simulink model "W04_4_inner_loop_offline"  (R2024b)
settings: Solver=ode4  StartTime=0.0  StopTime=40  FixedStep=0.05  RelTol=1e-3
values from neighbouring files (symbols this model uses):
  animate = 1    [W04_setup.m]
  Kd_psi = -400    [W04_setup.m]
  Ki_psi = 0    [W04_setup.m]
  Kp_psi = 800    [W04_setup.m]
  N_max = 500    [W04_setup.m]
  psi_ref_deg = 45    [W04_setup.m]
  use_ssa = 1    [W04_setup.m]
undefined symbols (not defined in the file or in its folder): DiscIntNeverNeededParam
libraries: slpidlib x1
settings Model: Creator=admin  LastModifiedBy=admin

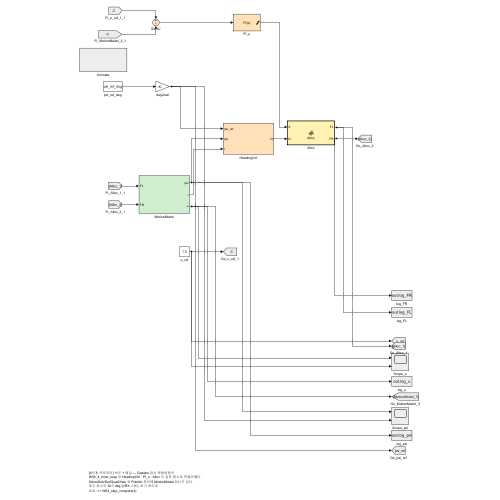
[thumbnail: Simulink's stored preview of the top-level diagram]
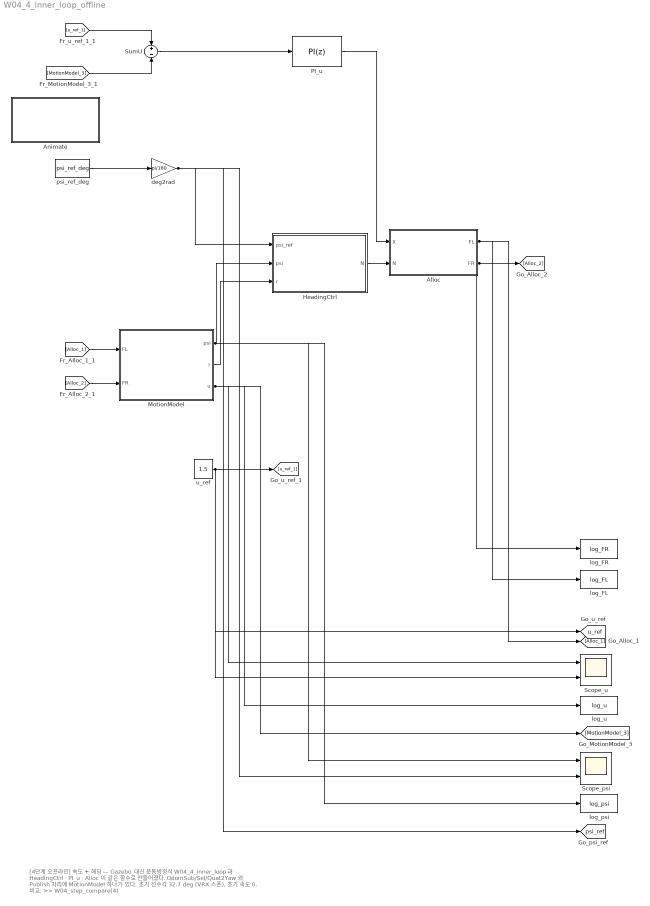
== system W04_4_inner_loop_offline ==
  note: [4단계 오프라인] 속도 + 헤딩 — Gazebo 대신 운동방정식
      | W04_4_inner_loop 과 HeadingCtrl · PI_u · Alloc 이 같은 함수로 만들어졌다.
      | OdomSub/Sel/Quat2Yaw 와 Publish 자리에 MotionModel 하나가 있다.
      | 초기 선수각 32.7 deg (VRX 스폰), 초기 속도 0.
      | 비교: >> W04_step_compare(4)
  Alloc : MATLAB Function  TreatAsAtomicUnit=on
  Animate : Subsystem
  HeadingCtrl : Subsystem
  MotionModel : Subsystem
  PI_u : slpidlib/PID Controller  Controller=PI  Form=Parallel  TimeDomain=Discrete-time  UseExternalTs=off  SampleTime=0.05  IntegratorMethod=Forward Euler  FilterMethod=Forward Euler  ControllerParametersSource=internal  P=300  I=40  UseKiTs=off  D=0  UseExternalDerivativeSource=off  N=100  UseFilter=on  TunerSelectOption=Transfer Function Based (PID Tuner App)  InitialConditionSource=internal  InitialConditionForIntegrator=0  InitialConditionForFilter=0  DifferentiatorICPrevScaledInput=0  ExternalReset=none  TrackingMode=off  Kt=1  LimitOutput=on  SatLimitsSource=internal  UpperSaturationLimit=500  LowerSaturationLimit=-500  LinearizeAsGain=off  AntiWindupMode=clamping  Kb=1  LimitIntegrator=off  UpperIntegratorSaturationLimit=inf  LowerIntegratorSaturationLimit=-inf  POutMin=[]  POutMax=[]  IOutMin=[]  IOutMax=[]  DOutMin=[]  DOutMax=[]  NOutMin=[]  NOutMax=[]  SumOutMin=[]  SumOutMax=[]  SaturationOutMin=[]  SaturationOutMax=[]  PParamMin=[]  PParamMax=[]  IParamMin=[]  IParamMax=[]  DParamMin=[]  DParamMax=[]  NParamMin=[]  NParamMax=[]  KbParamMin=[]  KbParamMax=[]  KtParamMin=[]  KtParamMax=[]  KbOutMin=[]  KbOutMax=[]  KtOutMin=[]  KtOutMax=[]  IntegratorOutMin=[]  IntegratorOutMax=[]  FilterOutMin=[]  FilterOutMax=[]  SumI1OutMin=[]  SumI1OutMax=[]  SumI2OutMin=[]  SumI2OutMax=[]  SumI3OutMin=[]  SumI3OutMax=[]  SumI4OutMin=[]  SumI4OutMax=[]  SumDOutMin=[]  SumDOutMax=[]  DifferentiatorOutMin=[]  DifferentiatorOutMax=[]  FilterDiffOutCoefMin=[]  FilterDiffOutCoefMax=[]  ReciprocalOutMin=[]  ReciprocalOutMax=[]  SumDenOutMin=[]  SumDenOutMax=[]  SumNumOutMin=[]  SumNumOutMax=[]  DivideOutMin=[]  DivideOutMax=[]  UdiffTsProdOutMin=[]  UdiffTsProdOutMax=[]  NTsProdOutMin=[]  NTsProdOutMax=[]  UintegralTsProdOutMin=[]  UintegralTsProdOutMax=[]  UngainTsProdOutMin=[]  UngainTsProdOutMax=[]  ClampingZeroOutDataTypeStr=Inherit: Inherit via back propagation  ClampingZeroOutMin=[]  ClampingZeroOutMax=[]  FilterDenConstantOutDataTypeStr=Inherit: Inherit via back propagation  FilterDenConstantOutMin=[]  FilterDenConstantOutMax=[]  PCopyOutDataTypeStr=Inherit: Inherit via back propagation  PCopyOutMin=[]  PCopyOutMax=[]  NCopyOutDataTypeStr=Inherit: Inherit via back propagation  NCopyOutMin=[]  NCopyOutMax=[]  IntegratorContinuousStateAttributes=''  IntegratorStateMustResolveToSignalObject=off  IntegratorRTWStateStorageClass=Auto  FilterContinuousStateAttributes=''  FilterStateMustResolveToSignalObject=off  FilterRTWStateStorageClass=Auto  ParallelPVariant=InternalParameters  IdealPVariant=Disabled  IVariant=InternalParameters  DVariant=Disabled  IntegratorVariant=Discrete  SatVariant=Enabled  AWVariant=DiscClampingParallel  PCopyVariant=Disabled  TRVariant=Disabled  FdbkBlocksVariant=Forward  IdealPFdbkVariant=Disabled  SatFdbkVariant=Disabled  DerivativeFilterVariant=Disabled  NVariant=Disabled  NCopyVariant=Disabled_SignalSpec  FilterICVariant=Disabled  IntegratorICVariant=InternalICs  ExternalResetVariant=Disabled  TRSumVariant=Passthrough  SumFdbkVariant=Disabled  SumVariant=Sum_PI  TsampFilterVariant=InternalTs  TsampNgainVariant=Passthrough  TsampIntegralVariant=Disabled_SignalSpec  ExternalSaturationOutDataTypeStr=Inherit: Same as second input  DerivativeSourceVariant=Disabled  PreIntVariant=InternalPreInt
      settings: LibrarySourceBlock=simulink/Discrete/Discrete PID Controller
  Scope_psi : Scope  NumInputPorts=2
  Scope_u : Scope  NumInputPorts=2
  SumU : Sum  Inputs=+-
  deg2rad : Gain  Gain=pi/180
  log_FL : ToWorkspace  VariableName=log_FL  SaveFormat=Timeseries  SampleTime=0.05
  log_FR : ToWorkspace  VariableName=log_FR  SaveFormat=Timeseries  SampleTime=0.05
  log_psi : ToWorkspace  VariableName=log_psi  SaveFormat=Timeseries  SampleTime=0.05
  log_u : ToWorkspace  VariableName=log_u  SaveFormat=Timeseries  SampleTime=0.05
  psi_ref_deg : Constant  Value=psi_ref_deg
  u_ref : Constant  Value=1.5
  tag scope: psi_ref=global, u_ref=global
  wires:
  [Alloc_2] -> MotionModel/2(FR)
  psi_ref_deg/1 -> deg2rad/1
  [u_ref_1] -> SumU/1
  SumU/1 -> PI_u/1
  [MotionModel_3] -> SumU/2
  [Alloc_1] -> MotionModel/1(FL)
  deg2rad/1 -> HeadingCtrl/1(psi_ref), [psi_ref], Scope_psi/2
  MotionModel/1(psi) -> HeadingCtrl/2(psi), Scope_psi/1, log_psi/1
  MotionModel/2(r) -> HeadingCtrl/3(r)
  PI_u/1 -> Alloc/1(X)
  HeadingCtrl/1(N) -> Alloc/2(N)
  Alloc/2(FR) -> [Alloc_2], log_FR/1
  Alloc/1(FL) -> log_FL/1, [Alloc_1]
  MotionModel/3(u) -> Scope_u/1, log_u/1, [MotionModel_3]
  u_ref/1 -> [u_ref], [u_ref_1], Scope_u/2

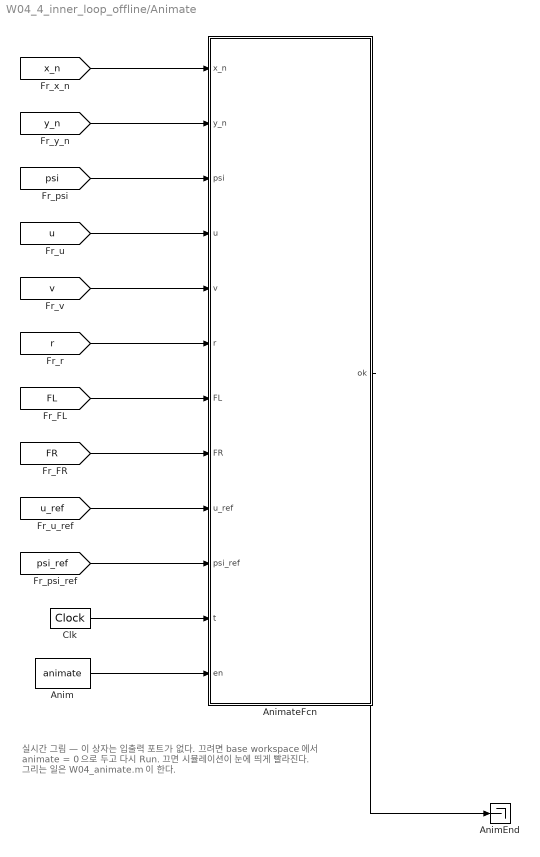
== system W04_4_inner_loop_offline/Animate ==
  note: 실시간 그림 — 이 상자는 입출력 포트가 없다.
      | 끄려면 base workspace 에서  animate = 0  으로 두고 다시 Run.
      | 끄면 시뮬레이션이 눈에 띄게 빨라진다.
      | 그리는 일은 W04_animate.m 이 한다.
  Anim : Constant  Value=animate
  AnimEnd : Terminator
  AnimateFcn : MATLAB Function  TreatAsAtomicUnit=on
  Clk : DigitalClock  SampleTime=0.05
  wires:
  [x_n] -> AnimateFcn/1(x_n)
  [y_n] -> AnimateFcn/2(y_n)
  [psi] -> AnimateFcn/3(psi)
  [u] -> AnimateFcn/4(u)
  [v] -> AnimateFcn/5(v)
  [r] -> AnimateFcn/6(r)
  [FL] -> AnimateFcn/7(FL)
  [FR] -> AnimateFcn/8(FR)
  [u_ref] -> AnimateFcn/9(u_ref)
  [psi_ref] -> AnimateFcn/10(psi_ref)
  Clk/1 -> AnimateFcn/11(t)
  Anim/1 -> AnimateFcn/12(en)
  AnimateFcn/1(ok) -> AnimEnd/1

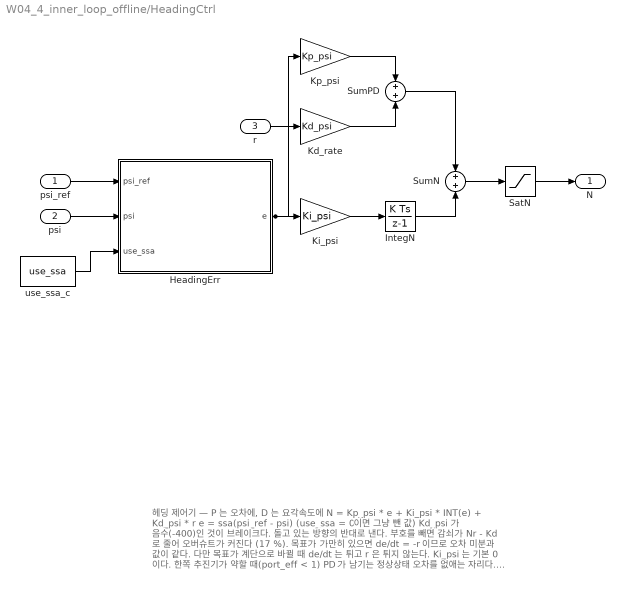
== system W04_4_inner_loop_offline/HeadingCtrl ==
  note: 헤딩 제어기 — P 는 오차에, D 는 요각속도에
      |
      |     N = Kp_psi * e  +  Ki_psi * INT(e)  +  Kd_psi * r
      |     e = ssa(psi_ref - psi)   (use_ssa = 0 이면 그냥 뺀 값)
      |
      | Kd_psi 가 음수(-400)인 것이 브레이크다. 돌고 있는 방향의 반대로 낸다.
      | 부호를 빼면 감쇠가 Nr - Kd 로 줄어 오버슈트가 커진다 (17 %).
      |
      | 목표가 가만히 있으면 de/dt = -r 이므로 오차 미분과 값이 같다.
      | 다만 목표가 계단으로 바뀔 때 de/dt 는 튀고 r 은 튀지 않는다.
      |
      | Ki_psi 는 기본 0 이다. 한쪽 추진기가 약할 때(port_eff < 1)
      | PD 가 남기는 정상상태 오차를 없애는 자리다.
      | 적분기에는 +-N_max 포화가 걸려 있다 (clamping 안티와인드업).
      |
      | 값은 전부 W04_setup.m — Kp_psi = 800, Kd_psi = -400.
      | 근거는 4주차 극배치 절과 W04_pole_place.m.
  psi_ref : Inport
  psi : Inport  Port=2
  r : Inport  Port=3
  HeadingErr : MATLAB Function  TreatAsAtomicUnit=on
  IntegN : DiscreteIntegrator  SampleTime=0.05  LimitOutput=on  UpperSaturationLimit=N_max  LowerSaturationLimit=-N_max  ICPrevOutput=DiscIntNeverNeededParam  ICPrevScaledInput=DiscIntNeverNeededParam
  Kd_rate : Gain  Gain=Kd_psi
  Ki_psi : Gain  Gain=Ki_psi
  Kp_psi : Gain  Gain=Kp_psi
  SatN : Saturate  UpperLimit=N_max  LowerLimit=-N_max
  SumN : Sum
  SumPD : Sum
  use_ssa_c : Constant  Value=use_ssa
  N : Outport
  wires:
  Kp_psi/1 -> SumPD/1
  psi_ref/1 -> HeadingErr/1(psi_ref)
  HeadingErr/1(e) -> Kp_psi/1, Ki_psi/1
  psi/1 -> HeadingErr/2(psi)
  use_ssa_c/1 -> HeadingErr/3(use_ssa)
  r/1 -> Kd_rate/1
  Kd_rate/1 -> SumPD/2
  Ki_psi/1 -> IntegN/1
  SumPD/1 -> SumN/1
  IntegN/1 -> SumN/2
  SumN/1 -> SatN/1
  SatN/1 -> N/1

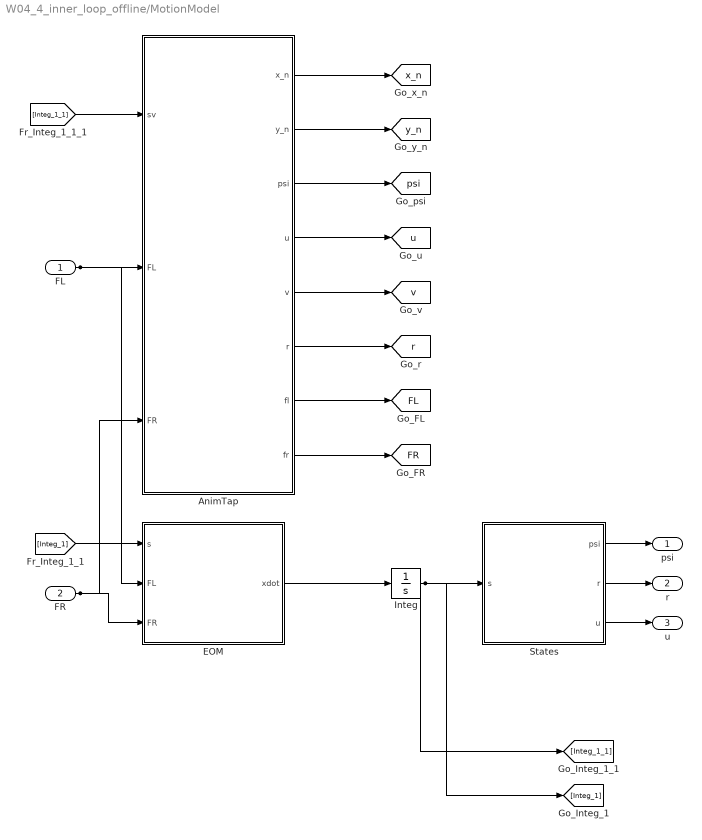
== system W04_4_inner_loop_offline/MotionModel ==
  FL : Inport
  FR : Inport  Port=2
  AnimTap : MATLAB Function  TreatAsAtomicUnit=on
  EOM : MATLAB Function  TreatAsAtomicUnit=on
  Integ : Integrator  InitialCondition=[0;0;0;0;0;32.7*pi/180]
  States : MATLAB Function  TreatAsAtomicUnit=on
  psi : Outport
  r : Outport  Port=2
  u : Outport  Port=3
  tag scope: FL=global, FR=global, psi=global, r=global, u=global, v=global, x_n=global, y_n=global
  wires:
  FL/1 -> EOM/2(FL), AnimTap/2(FL)
  [Integ_1_1] -> AnimTap/1(sv)
  AnimTap/4(u) -> [u]
  FR/1 -> EOM/3(FR), AnimTap/3(FR)
  [Integ_1] -> EOM/1(s)
  AnimTap/1(x_n) -> [x_n]
  AnimTap/2(y_n) -> [y_n]
  AnimTap/3(psi) -> [psi]
  AnimTap/6(r) -> [r]
  AnimTap/5(v) -> [v]
  AnimTap/8(fr) -> [FR]
  AnimTap/7(fl) -> [FL]
  EOM/1(xdot) -> Integ/1
  Integ/1 -> States/1(s), [Integ_1_1], [Integ_1]
  States/1(psi) -> psi/1
  States/2(r) -> r/1
  States/3(u) -> u/1

== matlab function W04_4_inner_loop_offline/MotionModel/States ==
  data: s input; psi output; r output; u output
function [psi, r, u] = States(s)
%#codegen
% Quat2Yaw 와 같은 출력 — 선수각은 [-pi, pi] 로 접는다
psi = atan2(sin(s(6)), cos(s(6)));
r = s(3);
u = s(1);

== matlab function W04_4_inner_loop_offline/MotionModel/EOM ==
  data: s input; xdot output; FL input; FR input
function xdot = EOM(s, FL, FR)
%#codegen
% 3-DOF WAM-V equations of motion, NED (3주차 1-8 절).
%   s = [u v r x_n y_n psi]'
m = 211;  Izz = 653;  Xu = 100;  Xuu = 150;  Yv = 100;  Yvv = 100;
Nr = 800;  Nrr = 800;  b_half = 1.027135;
u = s(1); v = s(2); r = s(3); psi = s(6);
X = FL + FR;
N = (FL - FR)*b_half;
du = (X - (Xu + Xuu*abs(u))*u)/m + v*r;
dv = (  - (Yv + Yvv*abs(v))*v)/m - u*r;
dr = (N - (Nr + Nrr*abs(r))*r)/Izz;
xdot = [du; dv; dr;
        u*cos(psi) - v*sin(psi);
        u*sin(psi) + v*cos(psi);
        r];

== matlab function W04_4_inner_loop_offline/MotionModel/AnimTap ==
  data: sv input; x_n output; FL input; FR input; y_n output; psi output; u output; v output; r output; fl output; fr output
function [x_n, y_n, psi, u, v, r, fl, fr] = AnimTap(sv, FL, FR)
%#codegen
% Display-only tap. sv = [u v r x_n y_n psi]'
x_n = sv(4);
y_n = sv(5);
psi = atan2(sin(sv(6)), cos(sv(6)));   % wrap to [-pi, pi]
u   = sv(1);
v   = sv(2);
r   = sv(3);
fl  = FL;
fr  = FR;

== matlab function W04_4_inner_loop_offline/HeadingCtrl/HeadingErr ==
  data: psi_ref input; e output; psi input; use_ssa input
function e = HeadingErr(psi_ref, psi, use_ssa)
%#codegen
% Heading error [rad].
d = psi_ref - psi;
if use_ssa >= 0.5
    % ssa : shortest signed angle, wrapped to (-pi, pi]
    e = atan2(sin(d), cos(d));
else
    % no wrap : 170 deg -> -170 deg becomes -340 deg, not +20 deg
    e = d;
end

== matlab function W04_4_inner_loop_offline/Alloc ==
  data: X input; FL output; N input; FR output
function [FL, FR] = Alloc(X, N)
%#codegen
% Differential thrust allocation for the 2-thruster WAM-V
%   X : surge force  [N]
%   N : yaw moment   [N*m], positive turns to starboard
B_half = 1.027135;      % half distance between thrusters [m]
Fmax   = 250;           % thrust limit per thruster [N]
FL = X/2 + N/(2*B_half);
FR = X/2 - N/(2*B_half);
FL = max(min(FL, Fmax), -Fmax);
FR = max(min(FR, Fmax), -Fmax);

== matlab function W04_4_inner_loop_offline/Animate/AnimateFcn ==
  data: x_n input; y_n input; psi input; u input; ok output; v input; r input; FL input; FR input; u_ref input; psi_ref input; t input; en input
function ok = AnimateFcn(x_n, y_n, psi, u, v, r, FL, FR, u_ref, psi_ref, t, en)
%#codegen
% 실시간 그림. MATLAB Function 블록은 그림을 그리지 못하므로 그리는 함수를
% extrinsic 으로 선언한다 — 코드를 만들지 않고 평범한 MATLAB 을 부른다.
% en = base workspace 의 animate (0 이면 그리지 않는다).
coder.extrinsic('W04_animate');
ok = 1;
if en > 0.5
    W04_animate(x_n, y_n, psi, u, v, r, FL, FR, u_ref, psi_ref, t);
end
